simulink model "K_error"  (R2017b)
settings: Solver=VariableStepAuto  StartTime=0.0  StopTime=10  RelTol=1e-3
libraries: simulink x1
settings Model: Creator=Cx001la  LastModifiedBy=Cx001la

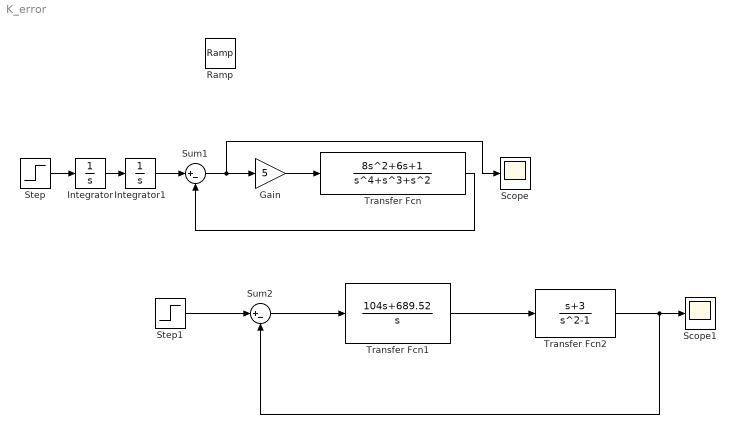
== system K_error ==
  Gain : Gain  Gain=5
  Integrator : Integrator
  Integrator1 : Integrator
  Ramp : simulink/Sources/Ramp  slope=1  start=0  X0=0
  Scope : Scope
  Scope1 : Scope
  Step : Step  SampleTime=0
  Step1 : Step  Time=0  SampleTime=0
  Sum1 : Sum  Inputs=|+-
  Sum2 : Sum  Inputs=|+-
  Transfer Fcn : TransferFcn  Numerator=[8 6 1]  Denominator=[1 1 1 0 0]
  Transfer Fcn1 : TransferFcn  Numerator=[104 689.52]  Denominator=[1 0]
  Transfer Fcn2 : TransferFcn  Numerator=[1 3]  Denominator=[1 0 -1]
  wires:
  Sum1/1 -> Scope/1, Gain/1
  Transfer Fcn/1 -> Sum1/2
  Gain/1 -> Transfer Fcn/1
  Step/1 -> Integrator/1
  Integrator/1 -> Integrator1/1
  Integrator1/1 -> Sum1/1
  Step1/1 -> Sum2/1
  Transfer Fcn2/1 -> Sum2/2, Scope1/1
  Sum2/1 -> Transfer Fcn1/1
  Transfer Fcn1/1 -> Transfer Fcn2/1
